simulink model "vehicle_control_system"  (R2024b)
settings: Solver=FixedStepAuto  StartTime=0.0  StopTime=12.0  FixedStep=0.05  RelTol=1e-3
PreLoadFcn:
  | addpath(genpath('C:\Users\megha\OneDrive\Pictures\Desktop\Matlab-simu'));
  | vp = vehicle_params();
  | cp = controller_params();
  | scenarios = generate_scenarios();
  | trajectory = scenarios.pothole_dodge;
  | control_mode = 'mpc';
settings Model: Creator=megha  LastModifiedBy=megha

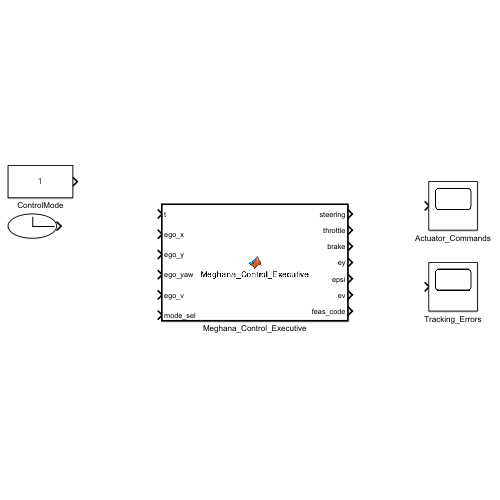
[thumbnail: Simulink's stored preview of the top-level diagram]
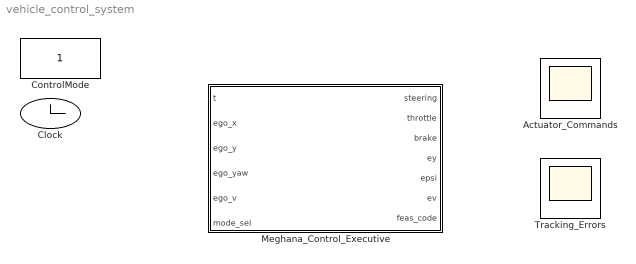
== system vehicle_control_system ==
  Actuator_Commands : Scope
  Clock : Clock
  ControlMode : Constant
  Meghana_Control_Executive : MATLAB Function  TreatAsAtomicUnit=on
  Tracking_Errors : Scope

== matlab function vehicle_control_system/Meghana_Control_Executive ==
  data: t input; steering output; ego_x input; ego_y input; ego_yaw input; ego_v input; mode_sel input; throttle output; brake output; ey output; epsi output; ev output; feas_code output
function [steering, throttle, brake, ey, epsi, ev, feas_code] = Meghana_Control_Executive(t, ego_x, ego_y, ego_yaw, ego_v, mode_sel)
% Master Controller Executive for SIH 26037
persistent vp cp traj internal_state safetyStatus;
if isempty(vp)
    vp = vehicle_params();
    cp = controller_params();
    sc = generate_scenarios();
    traj = sc.pothole_dodge;
    internal_state = [];
    safetyStatus = struct('safe','safe','TTC',99.0,'clearance',50.0,'reason','OK','emergency_flag',false);
end
modes = {'mpc', 'stanley', 'pure_pursuit'};
m_idx = max(1, min(3, round(mode_sel)));
ctrl_mode = modes{m_idx};
egoState = struct('timestamp', t, 'pose', [ego_x, ego_y, 0.0], 'velocity', [ego_v, 0.0, 0.0], 'heading', ego_yaw, 'covariance', eye(3));
[cmd, fb, internal_state] = vehicle_control_executive(traj, egoState, safetyStatus, ctrl_mode, internal_state, vp, cp);
steering = cmd.steering;
throttle = cmd.throttle;
brake = cmd.brake;
ey = fb.cross_track_err;
epsi = fb.heading_err;
ev = fb.speed_err;
feas_code = double(fb.feasibility_code);
end
